simulink model "PID_NL"  (R2020b)
settings: Solver=VariableStepAuto  StartTime=0.0  StopTime=20  RelTol=1e-3
values from neighbouring files (symbols this model uses):
  a0 = 0.001505    [params.m]
  a2 = -0.000055    (= -5.5e-05)    [params.m]
  alfa_o = 0    [params.m]
  g = 9.81    [params.m]
  I = m1*r1^2+m2*r2^2+m3*r3^2    (= 0.0018475)    [params.m]
  m1 = 0.031    [params.m]
  m2 = 0.019    [params.m]
  m3 = 0.02    [params.m]
  p1 = 0.052    [params.m]
  p2 = -0.0036    [params.m]
  r1 = 0.19    [params.m]
  r2 = 0.16    [params.m]
  r3 = 0.11    [params.m]
  vo = 3.855    [params.m]
libraries: pid_lib x1
settings Model: Creator=bou  LastModifiedBy=bou

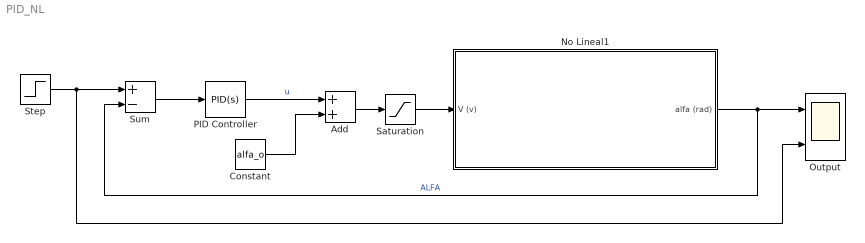
== system PID_NL ==
  Add : Sum
  Constant : Constant  Value=alfa_o
  No Lineal1 : Subsystem
  Output : Scope  NumInputPorts=2
  PID Controller : pid_lib/PID Controller  Controller=PID  Form=Parallel  TimeDomain=Continuous-time  UseExternalTs=off  SampleTime=-1  IntegratorMethod=Forward Euler  FilterMethod=Forward Euler  ControllerParametersSource=internal  P=0.0763  I=0.4638  D=1.2276  UseFilter=on  N=100  TunerSelectOption=Transfer Function Based (PID Tuner App)  InitialConditionSource=internal  InitialConditionForIntegrator=0  InitialConditionForFilter=0  DifferentiatorICPrevScaledInput=0  ExternalReset=none  TrackingMode=off  Kt=1  LimitOutput=off  SatLimitsSource=internal  UpperSaturationLimit=inf  LowerSaturationLimit=-inf  LinearizeAsGain=on  AntiWindupMode=none  Kb=1  POutMin=[]  POutMax=[]  IOutMin=[]  IOutMax=[]  DOutMin=[]  DOutMax=[]  NOutMin=[]  NOutMax=[]  SumOutMin=[]  SumOutMax=[]  SaturationOutMin=[]  SaturationOutMax=[]  PParamMin=[]  PParamMax=[]  IParamMin=[]  IParamMax=[]  DParamMin=[]  DParamMax=[]  NParamMin=[]  NParamMax=[]  KbParamMin=[]  KbParamMax=[]  KtParamMin=[]  KtParamMax=[]  KbOutMin=[]  KbOutMax=[]  KtOutMin=[]  KtOutMax=[]  IntegratorOutMin=[]  IntegratorOutMax=[]  FilterOutMin=[]  FilterOutMax=[]  SumI1OutMin=[]  SumI1OutMax=[]  SumI2OutMin=[]  SumI2OutMax=[]  SumI3OutMin=[]  SumI3OutMax=[]  SumI4OutMin=[]  SumI4OutMax=[]  SumDOutMin=[]  SumDOutMax=[]  DifferentiatorOutMin=[]  DifferentiatorOutMax=[]  FilterDiffOutCoefMin=[]  FilterDiffOutCoefMax=[]  ReciprocalOutMin=[]  ReciprocalOutMax=[]  SumDenOutMin=[]  SumDenOutMax=[]  SumNumOutMin=[]  SumNumOutMax=[]  DivideOutMin=[]  DivideOutMax=[]  UdiffTsProdOutMin=[]  UdiffTsProdOutMax=[]  NTsProdOutMin=[]  NTsProdOutMax=[]  UintegralTsProdOutMin=[]  UintegralTsProdOutMax=[]  UngainTsProdOutMin=[]  UngainTsProdOutMax=[]  IntegratorContinuousStateAttributes=''  IntegratorStateMustResolveToSignalObject=off  IntegratorRTWStateStorageClass=Auto  FilterContinuousStateAttributes=''  FilterStateMustResolveToSignalObject=off  FilterRTWStateStorageClass=Auto  ParallelPVariant=InternalParameters  IdealPVariant=Disabled  IVariant=InternalParameters  DVariant=InternalParameters  IntegratorVariant=Continuous  SatVariant=Disabled  AWVariant=Passthrough  PCopyVariant=Disabled  TRVariant=Disabled  FdbkBlocksVariant=Forward  IdealPFdbkVariant=Disabled  SatFdbkVariant=Disabled  DerivativeFilterVariant=ContFilter  NVariant=InternalParameters  NCopyVariant=Disabled  FilterICVariant=InternalICsFilter  IntegratorICVariant=InternalICs  ExternalResetVariant=Disabled  TRSumVariant=Passthrough  SumFdbkVariant=Disabled  SumVariant=Sum_PID  TsampFilterVariant=InternalTs  TsampNgainVariant=Passthrough  TsampIntegralVariant=Passthrough  ExternalSaturationOutDataTypeStr=Inherit: Same as second input
  Saturation : Saturate  UpperLimit=6.0  LowerLimit=0.0
  Step : Step  Time=0  Before=vo  After=vo+1  SampleTime=0
  Sum : Sum  Inputs=+-
  wires:
  Step/1 -> Sum/1, Output/2
  Saturation/1 -> No Lineal1/1(V (v))
  Add/1 -> Saturation/1
  Constant/1 -> Add/2
  No Lineal1/1(alfa (rad)) -> Output/1, Sum/2  "ALFA"
  Sum/1 -> PID Controller/1
  PID Controller/1 -> Add/1  "u"

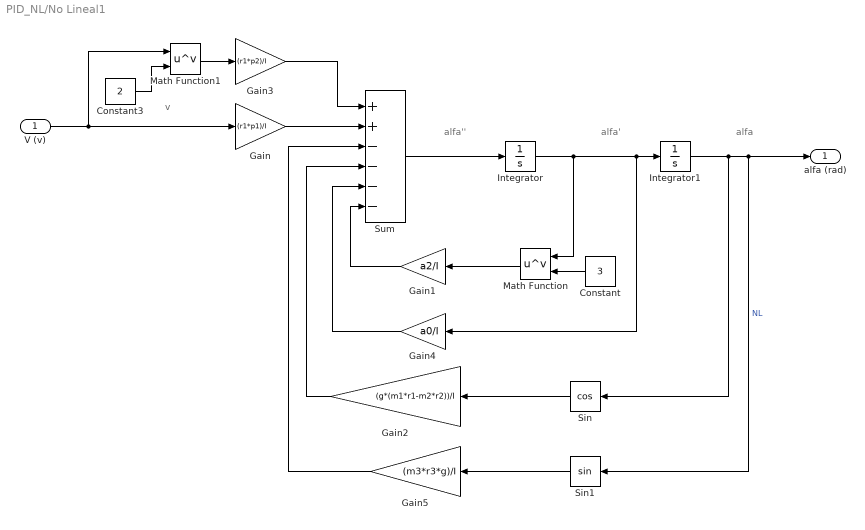
== system PID_NL/No Lineal1 ==
  note: v
  note: alfa
  note: alfa'
  note: alfa''
  V (v) : Inport
  Constant : Constant  Value=3
  Constant3 : Constant  Value=2
  Gain : Gain  Gain=(r1*p1)/I
  Gain1 : Gain  Gain=a2/I
  Gain2 : Gain  Gain=(g*(m1*r1-m2*r2))/I
  Gain3 : Gain  Gain=(r1*p2)/I
  Gain4 : Gain  Gain=a0/I
  Gain5 : Gain  Gain=(m3*r3*g)/I
  Integrator : Integrator  InitialCondition=alfa_o
  Integrator1 : Integrator  InitialCondition=alfa_o
  Math Function : Math  Operator=pow  SaturateOnIntegerOverflow=on
  Math Function1 : Math  Operator=pow  SaturateOnIntegerOverflow=on
  Sin : Trigonometry  Operator=cos
  Sin1 : Trigonometry
  Sum : Sum  Inputs=++----
  alfa (rad) : Outport
  wires:
  Sin/1 -> Gain2/1
  Gain5/1 -> Sum/3
  Constant3/1 -> Math Function1/2
  Integrator1/1 -> alfa (rad)/1, Sin1/1, Sin/1  "NL"
  Gain3/1 -> Sum/1
  Gain2/1 -> Sum/4
  V (v)/1 -> Math Function1/1, Gain/1
  Gain/1 -> Sum/2
  Sum/1 -> Integrator/1
  Sin1/1 -> Gain5/1
  Math Function1/1 -> Gain3/1
  Gain4/1 -> Sum/5
  Constant/1 -> Math Function/2
  Integrator/1 -> Integrator1/1, Gain4/1, Math Function/1
  Math Function/1 -> Gain1/1
  Gain1/1 -> Sum/6
